simulink model "BaseEngineController_LS_112"  (Simulink 7.7)
settings: Solver=FixedStepDiscrete  StartTime=0.0  StopTime=10.0  RelTol=1e-3
PreLoadFcn:
  | try, eval([bdroot '_setup']); catch, eval('model_setup', ''); end
InitFcn:
  | try, eval([bdroot '_setup']); catch, eval('model_setup', ''); end
undefined symbols (not defined in the file): ECM, H1, H2, High, motohawk_build_version, motohawk_trunc_name, motohawk_vardec_config_group, motohawk_vardec_path, True, xD
libraries: MotoHawk_lib x1417, motohawk_control_primitives_lib x183, motohawk_engine_lib x32, simulink x21, motohawk_annotations_lib x9, AutoDoc_lib x8, simulink_extras x4, motohawk_ccp_examples_lib x1, motohawk_control_primitives_motoshare_lib x1
(part 26 of 27)

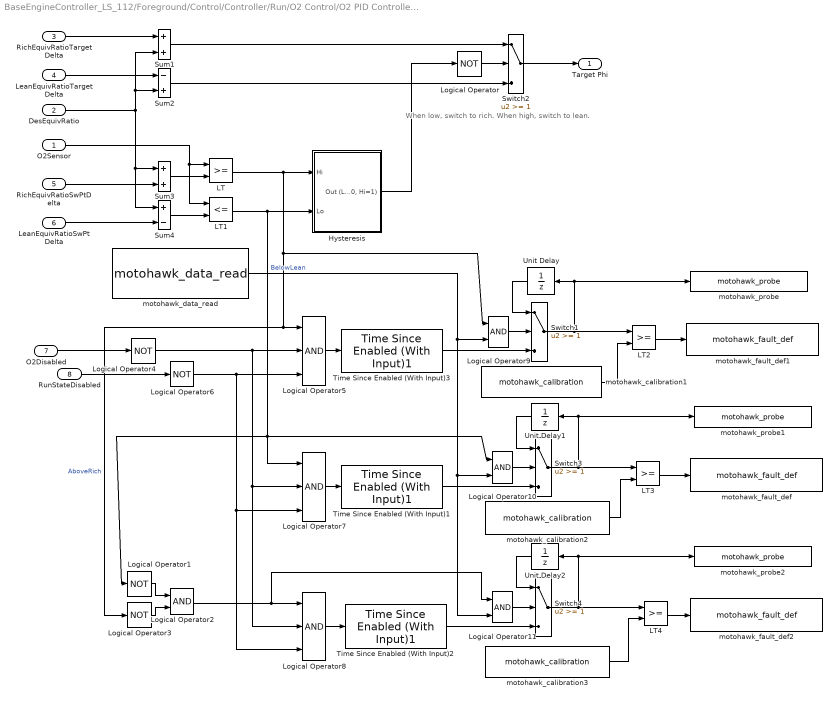
== system BaseEngineController_LS_112/Foreground/Control/Controller/Run/O2 Control/O2 PID Controller Bank A/Equivalence Ratio Perturbation ==
  note: When low, switch to rich.
      | When high, switch to lean.
  O2Sensor : Inport
  DesEquivRatio : Inport  Port=2
  RichEquivRatioTargetDelta : Inport  Port=3
  LeanEquivRatioTargetDelta : Inport  Port=4
  RichEquivRatioSwPtDelta : Inport  Port=5
  LeanEquivRatioSwPtDelta : Inport  Port=6
  O2Disabled : Inport  Port=7
  RunStateDisabled : Inport  Port=8
  Hysteresis : Subsystem
  LT{,2..4} (4 alike) : RelationalOperator  ZeroCross=off  InputSameDT=on
  LT1 : RelationalOperator  Operator=<=  ZeroCross=off  InputSameDT=on
  Logical Operator{,1,3..4,6} (5 alike) : Logic  Operator=NOT
  Logical Operator{2,9..11} (4 alike) : Logic
  Logical Operator5 : Logic  Inputs=3
  Logical Operator7 : Logic  Inputs=3
  Logical Operator8 : Logic  Inputs=3
  Sum1 : Sum  SaturateOnIntegerOverflow=on
  Sum2 : Sum  Inputs=-+  SaturateOnIntegerOverflow=on
  Sum3 : Sum  SaturateOnIntegerOverflow=on
  Sum4 : Sum  Inputs=+-  SaturateOnIntegerOverflow=on
  Switch{1..4} (4 alike) : Switch  Threshold=1  ZeroCross=off  InputSameDT=on
  Time Since Enabled (With Input)1 : motohawk_control_primitives_lib/Time Since Enabled (With Input)1  SystemSampleTime=-1  nam='O2LeanTimer_BankA'  samp_time=-1  init=0  upperlim=16000
  Time Since Enabled (With Input)2 : motohawk_control_primitives_lib/Time Since Enabled (With Input)1  SystemSampleTime=-1  nam='O2ActiveTimer_BankA'  samp_time=-1  init=0  upperlim=16000
  Time Since Enabled (With Input)3 : motohawk_control_primitives_lib/Time Since Enabled (With Input)1  SystemSampleTime=-1  nam='O2RichTimer_BankA'  samp_time=-1  init=0  upperlim=16000
  Unit Delay : UnitDelay  SampleTime=-1
  Unit Delay1 : UnitDelay  SampleTime=-1
  Unit Delay2 : UnitDelay  SampleTime=-1
  motohawk_calibration1 : MotoHawk_lib/Calibration & Probing Blocks/motohawk_calibration  nam='O2RichTimeThresh_BankA'  val=40  storage=Calibration  show_more=on  name_source=Use Parameter  data_type=Inherit from 'Default Value'  read_level=1  write_level=1  ovr_cals=on  view_as=Number  enum_struct={'Disabled', 'Enabled'}  vector_style=Wide Row  use_help_units=on  help='Time limit the O2 feedback can sit abovethe rich switch point before flagging O2FailedRich fault'  units='s'  use_header_enum=off  row_header_enum={}  col_header_enum={}  use_min_max=off  min_val=-inf  max_val=inf  use_precision=off  precision=''  gain=1  offset=0  exp=1  use_mototune_group=on  mototune_group=motohawk_vardec_path(gcb)
  motohawk_calibration2 : MotoHawk_lib/Calibration & Probing Blocks/motohawk_calibration  nam='O2LeanTimeThresh_BankA'  val=10  storage=Calibration  show_more=on  name_source=Use Parameter  data_type=Inherit from 'Default Value'  read_level=1  write_level=1  ovr_cals=on  view_as=Number  enum_struct={'Disabled', 'Enabled'}  vector_style=Wide Row  use_help_units=on  help='Time limit the O2 feedback can sit below the lean switch point before flagging O2FailedLean fault'  units='s'  use_header_enum=off  row_header_enum={}  col_header_enum={}  use_min_max=off  min_val=-inf  max_val=inf  use_precision=off  precision=''  gain=1  offset=0  exp=1  use_mototune_group=on  mototune_group=motohawk_vardec_path(gcb)
  motohawk_calibration3 : MotoHawk_lib/Calibration & Probing Blocks/motohawk_calibration  nam='O2ActiveTimeThresh_BankA'  val=40  storage=Calibration  show_more=on  name_source=Use Parameter  data_type=Inherit from 'Default Value'  read_level=1  write_level=1  ovr_cals=on  view_as=Number  enum_struct={'Disabled', 'Enabled'}  vector_style=Wide Row  use_help_units=on  help='Time limit O2 feedback can sit between rich and lean switch points before flagging O2NotActive fault'  units='s'  use_header_enum=off  row_header_enum={}  col_header_enum={}  use_min_max=off  min_val=-inf  max_val=inf  use_precision=off  precision=''  gain=1  offset=0  exp=1  use_mototune_group=on  mototune_group=motohawk_vardec_path(gcb)
  motohawk_data_read : MotoHawk_lib/Data Storage Blocks/motohawk_data_read  source=Lookup By Name  structure=Scalar  operation=Read scalar from location by index  sz_vec=4  sz_row=2  sz_col=3  typ=boolean  nam='DisableO2FaultAction'  checkNull=on  struct_inst_name='Struct1'  struct_nam='MyStruct'
  motohawk_fault_def : MotoHawk_lib/Fault Management Blocks/motohawk_fault_def  nam='O2FailedLean_BankA'  mode=Enabled  id=[]  x=25  y=50  input_suspected=on  indeterminate=off  increment_xy=on  downsample_count=1  ovr_cals=on  ovr_actions=on  show_actions=off  action1_name=''  action1_cond=(None)  action2_name=''  action2_cond=(None)  action3_name=''  action3_cond=(None)  action4_name=''  action4_cond=(None)
  motohawk_fault_def1 : MotoHawk_lib/Fault Management Blocks/motohawk_fault_def  nam='O2FailedRich_BankA'  mode=Enabled  id=[]  x=25  y=50  input_suspected=on  indeterminate=off  increment_xy=on  downsample_count=1  ovr_cals=on  ovr_actions=on  show_actions=off  action1_name=''  action1_cond=(None)  action2_name=''  action2_cond=(None)  action3_name=''  action3_cond=(None)  action4_name=''  action4_cond=(None)
  motohawk_fault_def2 : MotoHawk_lib/Fault Management Blocks/motohawk_fault_def  nam='O2NotActive_BankA'  mode=Enabled  id=[]  x=25  y=50  input_suspected=on  indeterminate=off  increment_xy=on  downsample_count=1  ovr_cals=on  ovr_actions=on  show_actions=off  action1_name=''  action1_cond=(None)  action2_name=''  action2_cond=(None)  action3_name=''  action3_cond=(None)  action4_name=''  action4_cond=(None)
  motohawk_probe : MotoHawk_lib/Calibration & Probing Blocks/motohawk_probe  nam='O2RichTime_BankA'  show_more=on  name_source=Use Parameter  read_level=1  view_as=Number  enum_struct={'Disabled', 'Enabled'}  vector_style=Wide Row  use_help_units=off  help=''  units=''  use_header_enum=off  row_header_enum={}  col_header_enum={}  use_precision=off  precision=''  gain=1  offset=0  exp=1  use_mototune_group=on  mototune_group=motohawk_vardec_path(gcb)
  motohawk_probe1 : MotoHawk_lib/Calibration & Probing Blocks/motohawk_probe  nam='O2LeanTime_BankA'  show_more=on  name_source=Use Parameter  read_level=1  view_as=Number  enum_struct={'Disabled', 'Enabled'}  vector_style=Wide Row  use_help_units=off  help=''  units=''  use_header_enum=off  row_header_enum={}  col_header_enum={}  use_precision=off  precision=''  gain=1  offset=0  exp=1  use_mototune_group=on  mototune_group=motohawk_vardec_path(gcb)
  motohawk_probe2 : MotoHawk_lib/Calibration & Probing Blocks/motohawk_probe  nam='O2NotActiveTime_BankA'  show_more=on  name_source=Use Parameter  read_level=1  view_as=Number  enum_struct={'Disabled', 'Enabled'}  vector_style=Wide Row  use_help_units=off  help=''  units=''  use_header_enum=off  row_header_enum={}  col_header_enum={}  use_precision=off  precision=''  gain=1  offset=0  exp=1  use_mototune_group=on  mototune_group=motohawk_vardec_path(gcb)
  Target Phi : Outport
  wires:
  Sum3/1 -> LT/2
  Sum4/1 -> LT1/2
  Switch2/1 -> Target Phi/1
  DesEquivRatio/1 -> Sum1/2, Sum2/2, Sum4/1, Sum3/1
  RichEquivRatioSwPtDelta/1 -> Sum3/2
  LeanEquivRatioSwPtDelta/1 -> Sum4/2
  Sum2/1 -> Switch2/3
  Sum1/1 -> Switch2/1
  LeanEquivRatioTargetDelta/1 -> Sum2/1
  RichEquivRatioTargetDelta/1 -> Sum1/1
  LT/1 -> Hysteresis/1(Hi), Logical Operator5/1, Logical Operator3/1, Logical Operator9/1  "AboveRich"
  LT1/1 -> Hysteresis/2(Lo), Logical Operator1/1, Logical Operator7/1, Logical Operator10/1  "BelowLean"
  Hysteresis/1("Out (Lo=0, Hi=1)") -> Logical Operator/1
  O2Sensor/1 -> LT1/1, LT/1
  Logical Operator/1 -> Switch2/2
  motohawk_calibration1/1 -> LT2/2
  LT2/1 -> motohawk_fault_def1/1
  LT3/1 -> motohawk_fault_def/1
  motohawk_calibration2/1 -> LT3/2
  LT4/1 -> motohawk_fault_def2/1
  motohawk_calibration3/1 -> LT4/2
  Logical Operator1/1 -> Logical Operator2/1
  Logical Operator3/1 -> Logical Operator2/2
  Logical Operator4/1 -> Logical Operator5/2, Logical Operator7/2, Logical Operator8/2
  O2Disabled/1 -> Logical Operator4/1
  RunStateDisabled/1 -> Logical Operator6/1
  Logical Operator6/1 -> Logical Operator5/3, Logical Operator7/3, Logical Operator8/3
  Logical Operator2/1 -> Logical Operator8/1, Logical Operator11/1
  Logical Operator5/1 -> Time Since Enabled (With Input)3/1
  Logical Operator7/1 -> Time Since Enabled (With Input)1/1
  Logical Operator8/1 -> Time Since Enabled (With Input)2/1
  Unit Delay/1 -> Switch1/1
  Time Since Enabled (With Input)3/1 -> Switch1/3
  Switch1/1 -> LT2/1, Unit Delay/1, motohawk_probe/1
  Logical Operator9/1 -> Switch1/2
  motohawk_data_read/1 -> Logical Operator9/2, Logical Operator10/2, Logical Operator11/2
  Unit Delay1/1 -> Switch3/1
  Switch3/1 -> LT3/1, Unit Delay1/1, motohawk_probe1/1
  Logical Operator10/1 -> Switch3/2
  Time Since Enabled (With Input)1/1 -> Switch3/3
  Unit Delay2/1 -> Switch4/1
  Switch4/1 -> LT4/1, Unit Delay2/1, motohawk_probe2/1
  Logical Operator11/1 -> Switch4/2
  Time Since Enabled (With Input)2/1 -> Switch4/3

== system BaseEngineController_LS_112/Foreground/Control/Controller/Run/O2 Control/O2 PID Controller Bank B/Closed-Loop O2 PID Controller ==
  O2Sensor : Inport
  TargetEquivRatio : Inport  Port=2
  ErrorGain : Inport  Port=3
  PGain : Inport  Port=4
  IGain : Inport  Port=5
  DGain : Inport  Port=6
  ITermUpperLimit : Inport  Port=7
  ITermLowerLimit : Inport  Port=8
  OutUpperLimit : Inport  Port=9
  OutLowerLimit : Inport  Port=10
  Reset : Inport  Port=11
  Constant : Constant  Value=0  OutDataTypeStr=Inherit: Inherit via back propagation
  Convert to Fuel Multiplier : Constant  OutDataTypeStr=Inherit: Inherit via back propagation
  Saturation : motohawk_control_primitives_lib/Saturation  SystemSampleTime=-1
  Sum : Sum  Inputs=++|  SaturateOnIntegerOverflow=on  InputSameDT=on
  Universal PID : motohawk_control_primitives_lib/Universal PID  Description=|  SystemSampleTime=-1  samp_time=.005
      | /* Name: ErrorGain Unit:mult ClassID:VAR StorageID:FLASH Access:RW4+RW3+NA2+NA1 TypeID:UINT4                   
      |    Gain:0.000000001 Min:0.000000000 Max:4.000000000 Format:10.9 UpdateID:REMOTE Help:"This gain is applied to "
      |    "the error term before it is used to calculate the P, I and D terms." VardecSig:6C */                       
      |                                                                                                                
      | /* Name: ITermLowerLim Unit:0 ClassID:VAR StorageID:FLASH Access:RW4+RW3+NA2+NA1 TypeID:SINT2 Gain:0.1         
      |    Min:-3276.8 Max:3276.7 Format:5.1 UpdateID:REMOTE Help:"Lower limit on the I-term value." VardecSig:6C */   
      |                                                                                                                
      | /* Name: ITermUpperLim ClassID:VAR StorageID:FLASH Access:RW4+RW3+NA2+NA1 TypeID:SINT2 Gain:0.1 Min:-3276.8    
      |    Max:3276.7 Format:5.1 UpdateID:REMOTE Help:"Upper limit on I-term value." VardecSig:6C */                   
      |                                                                                                                
      | /* Name: PIDOutLowerLim ClassID:VAR StorageID:FLASH Access:RW4+RW3+NA2+NA1 TypeID:SINT2 Gain:0.1               
      |    Min:-3276.8 Max:3276.7 Format:5.1 UpdateID:REMOTE Help:"Lower limit on PID output." VardecSig:6C */         
      |                                                                                                                
      | /* Name: PIDOutUpperLim ClassID:VAR StorageID:FLASH Access:RW4+RW3+NA2+NA1 TypeID:SINT2 Gain:0.1               
      |    Min:-3276.8 Max:3276.7 Format:3.1 UpdateID:REMOTE Help:"Upper limit on PID output." VardecSig:6C */
  motohawk_probe : MotoHawk_lib/Calibration & Probing Blocks/motohawk_probe  nam='LiquidO2Control_PTerm_BankB'  show_more=on  name_source=Use Parameter  read_level=1  view_as=Number  enum_struct={'Disabled', 'Enabled'}  vector_style=Wide Row  use_help_units=on  help='Closed-loop O2 control P-Term'  units='mult'  use_header_enum=off  row_header_enum={}  col_header_enum={}  use_precision=off  precision=''  gain=1  offset=0  exp=1  use_mototune_group=on  mototune_group=motohawk_vardec_path(gcb)
  motohawk_probe1 : MotoHawk_lib/Calibration & Probing Blocks/motohawk_probe  nam='LiquidO2Control_ITerm_BankB'  show_more=on  name_source=Use Parameter  read_level=1  view_as=Number  enum_struct={'Disabled', 'Enabled'}  vector_style=Wide Row  use_help_units=on  help='Closed-loop O2 control I-Term'  units='mult'  use_header_enum=off  row_header_enum={}  col_header_enum={}  use_precision=off  precision=''  gain=1  offset=0  exp=1  use_mototune_group=on  mototune_group=motohawk_vardec_path(gcb)
  motohawk_probe2 : MotoHawk_lib/Calibration & Probing Blocks/motohawk_probe  nam='LiquidO2Control_DTerm_BankB'  show_more=on  name_source=Use Parameter  read_level=1  view_as=Number  enum_struct={'Disabled', 'Enabled'}  vector_style=Wide Row  use_help_units=on  help='Closed-loop O2 control D-Term, for bank'  units='mult'  use_header_enum=off  row_header_enum={}  col_header_enum={}  use_precision=off  precision=''  gain=1  offset=0  exp=1  use_mototune_group=on  mototune_group=motohawk_vardec_path(gcb)
  motohawk_probe3 : MotoHawk_lib/Calibration & Probing Blocks/motohawk_probe  nam='LiquidO2Control_ErrorTerm_BankB'  show_more=on  name_source=Use Parameter  read_level=1  view_as=Number  enum_struct={'Disabled', 'Enabled'}  vector_style=Wide Row  use_help_units=on  help='Closed-loop O2 control error-term, for bank'  units='mult'  use_header_enum=off  row_header_enum={}  col_header_enum={}  use_precision=off  precision=''  gain=1  offset=0  exp=1  use_mototune_group=on  mototune_group=motohawk_vardec_path(gcb)
  Multiplier : Outport
  ITerm : Outport  Port=2
  wires:
  Reset/1 -> Universal PID/10
  Universal PID/3 -> motohawk_probe/1
  Universal PID/4 -> motohawk_probe1/1, ITerm/1
  Constant/1 -> Universal PID/7
  Universal PID/5 -> motohawk_probe2/1
  Saturation/1 -> Multiplier/1
  O2Sensor/1 -> Universal PID/1
  TargetEquivRatio/1 -> Universal PID/2
  ErrorGain/1 -> Universal PID/3
  PGain/1 -> Universal PID/4
  IGain/1 -> Universal PID/5
  DGain/1 -> Universal PID/6
  OutUpperLimit/1 -> Saturation/3
  Convert to Fuel Multiplier/1 -> Sum/1
  Universal PID/1 -> Sum/2
  Sum/1 -> Saturation/1
  ITermUpperLimit/1 -> Universal PID/9
  ITermLowerLimit/1 -> Universal PID/8
  OutLowerLimit/1 -> Saturation/2
  Universal PID/2 -> motohawk_probe3/1

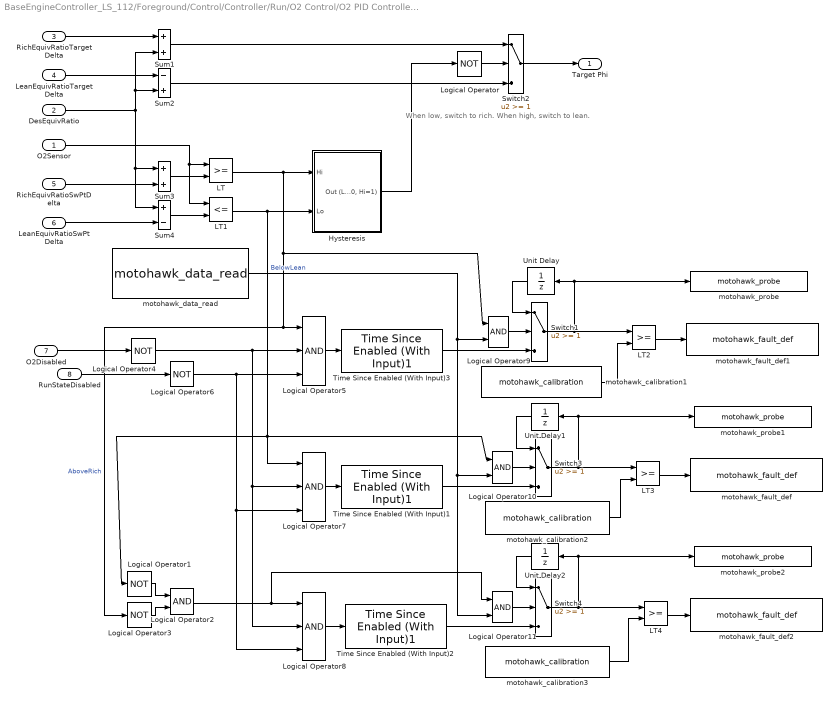
== system BaseEngineController_LS_112/Foreground/Control/Controller/Run/O2 Control/O2 PID Controller Bank B/Equivalence Ratio Perturbation ==
  note: When low, switch to rich.
      | When high, switch to lean.
  O2Sensor : Inport
  DesEquivRatio : Inport  Port=2
  RichEquivRatioTargetDelta : Inport  Port=3
  LeanEquivRatioTargetDelta : Inport  Port=4
  RichEquivRatioSwPtDelta : Inport  Port=5
  LeanEquivRatioSwPtDelta : Inport  Port=6
  O2Disabled : Inport  Port=7
  RunStateDisabled : Inport  Port=8
  Hysteresis : Subsystem
  LT{,2..4} (4 alike) : RelationalOperator  ZeroCross=off  InputSameDT=on
  LT1 : RelationalOperator  Operator=<=  ZeroCross=off  InputSameDT=on
  Logical Operator{,1,3..4,6} (5 alike) : Logic  Operator=NOT
  Logical Operator{2,9..11} (4 alike) : Logic
  Logical Operator5 : Logic  Inputs=3
  Logical Operator7 : Logic  Inputs=3
  Logical Operator8 : Logic  Inputs=3
  Sum1 : Sum  SaturateOnIntegerOverflow=on
  Sum2 : Sum  Inputs=-+  SaturateOnIntegerOverflow=on
  Sum3 : Sum  SaturateOnIntegerOverflow=on
  Sum4 : Sum  Inputs=+-  SaturateOnIntegerOverflow=on
  Switch{1..4} (4 alike) : Switch  Threshold=1  ZeroCross=off  InputSameDT=on
  Time Since Enabled (With Input)1 : motohawk_control_primitives_lib/Time Since Enabled (With Input)1  SystemSampleTime=-1  nam='O2LeanTimer_BankB'  samp_time=-1  init=0  upperlim=16000
  Time Since Enabled (With Input)2 : motohawk_control_primitives_lib/Time Since Enabled (With Input)1  SystemSampleTime=-1  nam='O2ActiveTimer_BankB'  samp_time=-1  init=0  upperlim=16000
  Time Since Enabled (With Input)3 : motohawk_control_primitives_lib/Time Since Enabled (With Input)1  SystemSampleTime=-1  nam='O2RichTimer_BankB'  samp_time=-1  init=0  upperlim=16000
  Unit Delay : UnitDelay  SampleTime=-1
  Unit Delay1 : UnitDelay  SampleTime=-1
  Unit Delay2 : UnitDelay  SampleTime=-1
  motohawk_calibration1 : MotoHawk_lib/Calibration & Probing Blocks/motohawk_calibration  nam='O2RichTimeThresh_BankB'  val=40  storage=Calibration  show_more=on  name_source=Use Parameter  data_type=Inherit from 'Default Value'  read_level=1  write_level=1  ovr_cals=on  view_as=Number  enum_struct={'Disabled', 'Enabled'}  vector_style=Wide Row  use_help_units=on  help='Time limit the O2 feedback can sit abovethe rich switch point before flagging O2FailedRich fault'  units='s'  use_header_enum=off  row_header_enum={}  col_header_enum={}  use_min_max=off  min_val=-inf  max_val=inf  use_precision=off  precision=''  gain=1  offset=0  exp=1  use_mototune_group=on  mototune_group=motohawk_vardec_path(gcb)
  motohawk_calibration2 : MotoHawk_lib/Calibration & Probing Blocks/motohawk_calibration  nam='O2LeanTimeThresh_BankB'  val=10  storage=Calibration  show_more=on  name_source=Use Parameter  data_type=Inherit from 'Default Value'  read_level=1  write_level=1  ovr_cals=on  view_as=Number  enum_struct={'Disabled', 'Enabled'}  vector_style=Wide Row  use_help_units=on  help='Time limit the O2 feedback can sit below the lean switch point before flagging O2FailedLean fault'  units='s'  use_header_enum=off  row_header_enum={}  col_header_enum={}  use_min_max=off  min_val=-inf  max_val=inf  use_precision=off  precision=''  gain=1  offset=0  exp=1  use_mototune_group=on  mototune_group=motohawk_vardec_path(gcb)
  motohawk_calibration3 : MotoHawk_lib/Calibration & Probing Blocks/motohawk_calibration  nam='O2ActiveTimeThresh_BankB'  val=40  storage=Calibration  show_more=on  name_source=Use Parameter  data_type=Inherit from 'Default Value'  read_level=1  write_level=1  ovr_cals=on  view_as=Number  enum_struct={'Disabled', 'Enabled'}  vector_style=Wide Row  use_help_units=on  help='Time limit O2 feedback can sit between rich and lean switch points before flagging O2NotActive fault'  units='s'  use_header_enum=off  row_header_enum={}  col_header_enum={}  use_min_max=off  min_val=-inf  max_val=inf  use_precision=off  precision=''  gain=1  offset=0  exp=1  use_mototune_group=on  mototune_group=motohawk_vardec_path(gcb)
  motohawk_data_read : MotoHawk_lib/Data Storage Blocks/motohawk_data_read  source=Lookup By Name  structure=Scalar  operation=Read scalar from location by index  sz_vec=4  sz_row=2  sz_col=3  typ=boolean  nam='DisableO2FaultAction'  checkNull=on  struct_inst_name='Struct1'  struct_nam='MyStruct'
  motohawk_fault_def : MotoHawk_lib/Fault Management Blocks/motohawk_fault_def  nam='O2FailedLean_BankB'  mode=Enabled  id=[]  x=25  y=50  input_suspected=on  indeterminate=off  increment_xy=on  downsample_count=1  ovr_cals=on  ovr_actions=on  show_actions=off  action1_name=''  action1_cond=(None)  action2_name=''  action2_cond=(None)  action3_name=''  action3_cond=(None)  action4_name=''  action4_cond=(None)
  motohawk_fault_def1 : MotoHawk_lib/Fault Management Blocks/motohawk_fault_def  nam='O2FailedRich_BankB'  mode=Enabled  id=[]  x=25  y=50  input_suspected=on  indeterminate=off  increment_xy=on  downsample_count=1  ovr_cals=on  ovr_actions=on  show_actions=off  action1_name=''  action1_cond=(None)  action2_name=''  action2_cond=(None)  action3_name=''  action3_cond=(None)  action4_name=''  action4_cond=(None)
  motohawk_fault_def2 : MotoHawk_lib/Fault Management Blocks/motohawk_fault_def  nam='O2NotActive_BankB'  mode=Enabled  id=[]  x=25  y=50  input_suspected=on  indeterminate=off  increment_xy=on  downsample_count=1  ovr_cals=on  ovr_actions=on  show_actions=off  action1_name=''  action1_cond=(None)  action2_name=''  action2_cond=(None)  action3_name=''  action3_cond=(None)  action4_name=''  action4_cond=(None)
  motohawk_probe : MotoHawk_lib/Calibration & Probing Blocks/motohawk_probe  nam='O2RichTime_BankB'  show_more=on  name_source=Use Parameter  read_level=1  view_as=Number  enum_struct={'Disabled', 'Enabled'}  vector_style=Wide Row  use_help_units=off  help=''  units=''  use_header_enum=off  row_header_enum={}  col_header_enum={}  use_precision=off  precision=''  gain=1  offset=0  exp=1  use_mototune_group=on  mototune_group=motohawk_vardec_path(gcb)
  motohawk_probe1 : MotoHawk_lib/Calibration & Probing Blocks/motohawk_probe  nam='O2LeanTime_BankB'  show_more=on  name_source=Use Parameter  read_level=1  view_as=Number  enum_struct={'Disabled', 'Enabled'}  vector_style=Wide Row  use_help_units=off  help=''  units=''  use_header_enum=off  row_header_enum={}  col_header_enum={}  use_precision=off  precision=''  gain=1  offset=0  exp=1  use_mototune_group=on  mototune_group=motohawk_vardec_path(gcb)
  motohawk_probe2 : MotoHawk_lib/Calibration & Probing Blocks/motohawk_probe  nam='O2NotActiveTime_BankB'  show_more=on  name_source=Use Parameter  read_level=1  view_as=Number  enum_struct={'Disabled', 'Enabled'}  vector_style=Wide Row  use_help_units=off  help=''  units=''  use_header_enum=off  row_header_enum={}  col_header_enum={}  use_precision=off  precision=''  gain=1  offset=0  exp=1  use_mototune_group=on  mototune_group=motohawk_vardec_path(gcb)
  Target Phi : Outport
  wires:
  Sum3/1 -> LT/2
  Sum4/1 -> LT1/2
  Switch2/1 -> Target Phi/1
  DesEquivRatio/1 -> Sum1/2, Sum2/2, Sum4/1, Sum3/1
  RichEquivRatioSwPtDelta/1 -> Sum3/2
  LeanEquivRatioSwPtDelta/1 -> Sum4/2
  Sum2/1 -> Switch2/3
  Sum1/1 -> Switch2/1
  LeanEquivRatioTargetDelta/1 -> Sum2/1
  RichEquivRatioTargetDelta/1 -> Sum1/1
  LT/1 -> Hysteresis/1(Hi), Logical Operator5/1, Logical Operator3/1, Logical Operator9/1  "AboveRich"
  LT1/1 -> Hysteresis/2(Lo), Logical Operator1/1, Logical Operator7/1, Logical Operator10/1  "BelowLean"
  Hysteresis/1("Out (Lo=0, Hi=1)") -> Logical Operator/1
  O2Sensor/1 -> LT1/1, LT/1
  Logical Operator/1 -> Switch2/2
  motohawk_calibration1/1 -> LT2/2
  LT2/1 -> motohawk_fault_def1/1
  LT3/1 -> motohawk_fault_def/1
  motohawk_calibration2/1 -> LT3/2
  LT4/1 -> motohawk_fault_def2/1
  motohawk_calibration3/1 -> LT4/2
  Logical Operator1/1 -> Logical Operator2/1
  Logical Operator3/1 -> Logical Operator2/2
  Logical Operator4/1 -> Logical Operator5/2, Logical Operator7/2, Logical Operator8/2
  O2Disabled/1 -> Logical Operator4/1
  RunStateDisabled/1 -> Logical Operator6/1
  Logical Operator6/1 -> Logical Operator5/3, Logical Operator7/3, Logical Operator8/3
  Logical Operator2/1 -> Logical Operator8/1, Logical Operator11/1
  Logical Operator5/1 -> Time Since Enabled (With Input)3/1
  Logical Operator7/1 -> Time Since Enabled (With Input)1/1
  Logical Operator8/1 -> Time Since Enabled (With Input)2/1
  Unit Delay/1 -> Switch1/1
  Time Since Enabled (With Input)3/1 -> Switch1/3
  Switch1/1 -> LT2/1, Unit Delay/1, motohawk_probe/1
  Logical Operator9/1 -> Switch1/2
  motohawk_data_read/1 -> Logical Operator9/2, Logical Operator10/2, Logical Operator11/2
  Unit Delay1/1 -> Switch3/1
  Switch3/1 -> LT3/1, Unit Delay1/1, motohawk_probe1/1
  Logical Operator10/1 -> Switch3/2
  Time Since Enabled (With Input)1/1 -> Switch3/3
  Unit Delay2/1 -> Switch4/1
  Switch4/1 -> LT4/1, Unit Delay2/1, motohawk_probe2/1
  Logical Operator11/1 -> Switch4/2
  Time Since Enabled (With Input)2/1 -> Switch4/3

== system BaseEngineController_LS_112/Foreground/Control/Controller/Stall/FAN Control/Hysterisis/Hysteresis ==
  note: Hi & !Lo => Hi
      | Lo & !Hi => Lo
      | Otherwise, Hold
  Hi : Inport
  Lo : Inport  Port=2
  Combinatorial  Logic : CombinatorialLogic  TruthTable=[0 0;0 1;1 1;0 0]
  Demux : Demux  Outputs=2
  Mux : Mux  Inputs=2
  Switch1 : Switch  Threshold=0.5  SaturateOnIntegerOverflow=on  InputSameDT=on
  Unit Delay : UnitDelay  SampleTime=-1
  "Out (Lo=0, Hi=1)" : Outport
  wires:
  Mux/1 -> Combinatorial  Logic/1
  Combinatorial  Logic/1 -> Demux/1
  Demux/1 -> Switch1/1
  Demux/2 -> Switch1/2
  Unit Delay/1 -> Switch1/3
  Switch1/1 -> Unit Delay/1, "Out (Lo=0, Hi=1)"/1
  Hi/1 -> Mux/1
  Lo/1 -> Mux/2

== system BaseEngineController_LS_112/Foreground/Control/Controller/Stall/FAN Control/Hysterisis1/Hysteresis ==
  note: Hi & !Lo => Hi
      | Lo & !Hi => Lo
      | Otherwise, Hold
  Hi : Inport
  Lo : Inport  Port=2
  Combinatorial  Logic : CombinatorialLogic  TruthTable=[0 0;0 1;1 1;0 0]
  Demux : Demux  Outputs=2
  Mux : Mux  Inputs=2
  Switch1 : Switch  Threshold=0.5  SaturateOnIntegerOverflow=on  InputSameDT=on
  Unit Delay : UnitDelay  SampleTime=-1
  "Out (Lo=0, Hi=1)" : Outport
  wires:
  Mux/1 -> Combinatorial  Logic/1
  Combinatorial  Logic/1 -> Demux/1
  Demux/1 -> Switch1/1
  Demux/2 -> Switch1/2
  Unit Delay/1 -> Switch1/3
  Switch1/1 -> Unit Delay/1, "Out (Lo=0, Hi=1)"/1
  Hi/1 -> Mux/1
  Lo/1 -> Mux/2

== system BaseEngineController_LS_112/Foreground/Control/Controller/Stall/FAN Control/Hysterisis2/Hysteresis ==
  note: Hi & !Lo => Hi
      | Lo & !Hi => Lo
      | Otherwise, Hold
  Hi : Inport
  Lo : Inport  Port=2
  Combinatorial  Logic : CombinatorialLogic  TruthTable=[0 0;0 1;1 1;0 0]
  Demux : Demux  Outputs=2
  Mux : Mux  Inputs=2
  Switch1 : Switch  Threshold=0.5  SaturateOnIntegerOverflow=on  InputSameDT=on
  Unit Delay : UnitDelay  SampleTime=-1
  "Out (Lo=0, Hi=1)" : Outport
  wires:
  Mux/1 -> Combinatorial  Logic/1
  Combinatorial  Logic/1 -> Demux/1
  Demux/1 -> Switch1/1
  Demux/2 -> Switch1/2
  Unit Delay/1 -> Switch1/3
  Switch1/1 -> Unit Delay/1, "Out (Lo=0, Hi=1)"/1
  Hi/1 -> Mux/1
  Lo/1 -> Mux/2

== system BaseEngineController_LS_112/Foreground/Control/Diagnostics/MISFIRE/MisfireDiagSub/MisfireDiagFunc/DetermineMisfire ==
  Compare To Constant : simulink/Logic and Bit Operations/Compare To Constant  SystemSampleTime=-1  relop=>  const=0  LogicOutDataTypeMode=uint8
  DetermineCylinder : Subsystem
  Logical Operator1 : Logic  AllPortsSameDT=off  OutDataTypeStr=boolean
  Product : Product  RndMeth=Zero
  Relational Operator1 : RelationalOperator  Operator=<=  OutDataTypeStr=boolean
  Rising Edge : motohawk_control_primitives_lib/Rising Edge  SystemSampleTime=-1
  SetHardFault : Subsystem
  Sum : Sum  Inputs=|+-
  motohawk_calibration1 : MotoHawk_lib/Calibration & Probing Blocks/motohawk_calibration  nam='MisfireDiag_HardMisfireThreshold'  val=50  storage=Calibration  show_more=off  name_source=Use Parameter  data_type=Inherit from 'Default Value'  read_level=1  write_level=1  ovr_cals=on  view_as=Number  enum_struct={'Disabled', 'Enabled'}  vector_style=Wide Row  use_help_units=off  help=''  units=''  use_header_enum=off  row_header_enum={}  col_header_enum={}  use_min_max=off  min_val=-inf  max_val=inf  use_precision=off  precision=''  gain=1  offset=0  exp=1  use_mototune_group=off  mototune_group=motohawk_vardec_path(gcb)
  motohawk_data_read : MotoHawk_lib/Data Storage Blocks/motohawk_data_read  source=Lookup By Name  structure=Vector  operation=Read scalar from location by index  sz_vec=8  sz_row=2  sz_col=3  typ=uint16  nam='MisfireDiag_StartRPM'  checkNull=on  struct_inst_name='MyData'  struct_nam='MyStruct'
  motohawk_data_read1 : MotoHawk_lib/Data Storage Blocks/motohawk_data_read  source=Lookup By Name  structure=Vector  operation=Read scalar from location by index  sz_vec=8  sz_row=2  sz_col=3  typ=uint16  nam='MisfireDiag_StopRPM'  checkNull=on  struct_inst_name='MyData'  struct_nam='MyStruct'
  motohawk_data_read2 : MotoHawk_lib/Data Storage Blocks/motohawk_data_read  source=Lookup By Name  structure=Vector  operation=Read entire data structure at once  sz_vec=8  sz_row=2  sz_col=3  typ=boolean  nam='MisfireDiag_RPMDR'  checkNull=on  struct_inst_name='MyData'  struct_nam='MyStruct'
  wires:
  motohawk_data_read2/1 -> Rising Edge/1
  Sum/1 -> [RPMDelta]
  motohawk_data_read1/1 -> Sum/1
  motohawk_data_read/1 -> Sum/2
  [RPMDelta] -> Relational Operator1/1
  motohawk_calibration1/1 -> Relational Operator1/2
  Rising Edge/1 -> [RPMDR_Rising]
  Logical Operator1/1 -> Product/2
  [RPMDR_Rising] -> DetermineCylinder/1(ArrayIn)
  DetermineCylinder/1(CylinderNum) -> motohawk_data_read1/1, motohawk_data_read/1, Compare To Constant/1, Product/1
  Relational Operator1/1 -> Logical Operator1/1
  Compare To Constant/1 -> Logical Operator1/2
  Product/1 -> SetHardFault/1(CylNum)

== system BaseEngineController_LS_112/Foreground/Control/Diagnostics/MISFIRE/MisfireDiagSub/MisfireDiagFunc/StoreRPMData ==
  DetermineCylinder : Subsystem
  DetermineCylinder1 : Subsystem
  EncoderAngleArb : Subsystem
  Gain : Gain  Gain=16
  Gain1 : Gain  Gain=16
  LatchForAverage : Subsystem
  LatchForAverage1 : Subsystem
  Logical Operator : Logic  AllPortsSameDT=off  OutDataTypeStr=boolean
  Logical Operator1 : Logic  AllPortsSameDT=off  OutDataTypeStr=boolean
  Logical Operator2 : Logic  Operator=OR  Inputs=1  AllPortsSameDT=off  OutDataTypeStr=boolean
  Logical Operator3 : Logic  Operator=OR  Inputs=1  AllPortsSameDT=off  OutDataTypeStr=boolean
  Relational Operator : RelationalOperator  Operator=<=  OutDataTypeStr=boolean
  Relational Operator1 : RelationalOperator  OutDataTypeStr=boolean
  Relational Operator2 : RelationalOperator  Operator=<=  OutDataTypeStr=boolean
  Relational Operator3 : RelationalOperator  OutDataTypeStr=boolean
  StoreRPMStart : Subsystem  TreatAsAtomicUnit=on
  StoreRPMStart1 : Subsystem  TreatAsAtomicUnit=on
  Sum : Sum  Inputs=|++
  Sum1 : Sum  Inputs=+-|
  Sum2 : Sum  Inputs=|++
  Sum3 : Sum  Inputs=+-|
  motohawk_calibration : MotoHawk_lib/Calibration & Probing Blocks/motohawk_calibration  nam='MisfireDiag_StartAngles'  val=[0,0,0,0,0,0,0,0]  storage=Calibration  show_more=on  name_source=Use Parameter  data_type=uint16  read_level=1  write_level=1  ovr_cals=on  view_as=Number  enum_struct={'Disabled', 'Enabled'}  vector_style=Wide Row  use_help_units=off  help=''  units=''  use_header_enum=off  row_header_enum={}  col_header_enum={}  use_min_max=off  min_val=-inf  max_val=inf  use_precision=off  precision=''  gain=1  offset=0  exp=1  use_mototune_group=off  mototune_group=motohawk_vardec_path(gcb)
  motohawk_calibration1 : MotoHawk_lib/Calibration & Probing Blocks/motohawk_calibration  nam='MisfireDiag_StopAngles'  val=[0,0,0,0,0,0,0,0]  storage=Calibration  show_more=on  name_source=Use Parameter  data_type=uint16  read_level=1  write_level=1  ovr_cals=on  view_as=Number  enum_struct={'Disabled', 'Enabled'}  vector_style=Wide Row  use_help_units=off  help=''  units=''  use_header_enum=off  row_header_enum={}  col_header_enum={}  use_min_max=off  min_val=-inf  max_val=inf  use_precision=off  precision=''  gain=1  offset=0  exp=1  use_mototune_group=off  mototune_group=motohawk_vardec_path(gcb)
  motohawk_calibration2 : MotoHawk_lib/Calibration & Probing Blocks/motohawk_calibration  nam='MisfireDiag_AngleHyst'  val=4  storage=Calibration  show_more=on  name_source=Use Parameter  data_type=uint16  read_level=1  write_level=1  ovr_cals=on  view_as=Number  enum_struct={'Disabled', 'Enabled'}  vector_style=Wide Row  use_help_units=off  help=''  units=''  use_header_enum=off  row_header_enum={}  col_header_enum={}  use_min_max=off  min_val=-inf  max_val=inf  use_precision=off  precision=''  gain=1  offset=0  exp=1  use_mototune_group=off  mototune_group=motohawk_vardec_path(gcb)
  motohawk_probe : MotoHawk_lib/Calibration & Probing Blocks/motohawk_probe  nam='MisfireDiag_EncoderAngle'  show_more=off  name_source=Use Parameter  read_level=1  view_as=Number  enum_struct={'Disabled', 'Enabled'}  vector_style=Wide Row  use_help_units=off  help=''  units=''  use_header_enum=off  row_header_enum={}  col_header_enum={}  use_precision=off  precision=''  gain=1  offset=0  exp=1  use_mototune_group=off  mototune_group=motohawk_vardec_path(gcb)
  motohawk_probe3 : MotoHawk_lib/Calibration & Probing Blocks/motohawk_probe  nam='MisfireDiag_AverageStartRPMDR'  show_more=off  name_source=Use Parameter  read_level=1  view_as=Number  enum_struct={'Disabled', 'Enabled'}  vector_style=Wide Row  use_help_units=off  help=''  units=''  use_header_enum=off  row_header_enum={}  col_header_enum={}  use_precision=off  precision=''  gain=1  offset=0  exp=1  use_mototune_group=off  mototune_group=motohawk_vardec_path(gcb)
  motohawk_probe4 : MotoHawk_lib/Calibration & Probing Blocks/motohawk_probe  nam='MisfireDiag_AverageStartRPM'  show_more=off  name_source=Use Parameter  read_level=1  view_as=Number  enum_struct={'Disabled', 'Enabled'}  vector_style=Wide Row  use_help_units=off  help=''  units=''  use_header_enum=off  row_header_enum={}  col_header_enum={}  use_precision=off  precision=''  gain=1  offset=0  exp=1  use_mototune_group=off  mototune_group=motohawk_vardec_path(gcb)
  motohawk_probe5 : MotoHawk_lib/Calibration & Probing Blocks/motohawk_probe  nam='MisfireDiag_AverageStopRPMDR'  show_more=off  name_source=Use Parameter  read_level=1  view_as=Number  enum_struct={'Disabled', 'Enabled'}  vector_style=Wide Row  use_help_units=off  help=''  units=''  use_header_enum=off  row_header_enum={}  col_header_enum={}  use_precision=off  precision=''  gain=1  offset=0  exp=1  use_mototune_group=off  mototune_group=motohawk_vardec_path(gcb)
  motohawk_probe6 : MotoHawk_lib/Calibration & Probing Blocks/motohawk_probe  nam='MisfireDiag_AverageStopRPM'  show_more=off  name_source=Use Parameter  read_level=1  view_as=Number  enum_struct={'Disabled', 'Enabled'}  vector_style=Wide Row  use_help_units=off  help=''  units=''  use_header_enum=off  row_header_enum={}  col_header_enum={}  use_precision=off  precision=''  gain=1  offset=0  exp=1  use_mototune_group=off  mototune_group=motohawk_vardec_path(gcb)
  wires:
  motohawk_calibration/1 -> Gain/1
  EncoderAngleArb/1(EncoderAngle_116) -> [EncoderAngle], motohawk_probe/1
  motohawk_calibration2/1 -> [EncoderAngleHyst]
  Gain/1 -> Sum1/1, Sum/2
  [EncoderAngleHyst] -> Sum/1
  [EncoderAngleHyst] -> Sum1/2
  Sum/1 -> Relational Operator/1
  Sum1/1 -> Relational Operator1/1
  [EncoderAngle] -> Relational Operator/2
  [EncoderAngle] -> Relational Operator1/2
  Relational Operator1/1 -> Logical Operator/2
  Relational Operator/1 -> Logical Operator/1
  Gain1/1 -> Sum3/1, Sum2/2
  [EncoderAngleHyst] -> Sum2/1
  [EncoderAngleHyst] -> Sum3/2
  Sum2/1 -> Relational Operator2/1
  Sum3/1 -> Relational Operator3/1
  [EncoderAngle] -> Relational Operator2/2
  [EncoderAngle] -> Relational Operator3/2
  Relational Operator3/1 -> Logical Operator1/2
  Relational Operator2/1 -> Logical Operator1/1
  motohawk_calibration1/1 -> Gain1/1
  Logical Operator/1 -> Logical Operator2/1, DetermineCylinder/1(ArrayIn)
  Logical Operator1/1 -> Logical Operator3/1, DetermineCylinder1/1(ArrayIn)
  Logical Operator2/1 -> LatchForAverage/1(Enbl)
  DetermineCylinder/1(CylinderNum) -> StoreRPMStart/2(CylinderNum)
  LatchForAverage/1(AverageRPMDR) -> StoreRPMStart/Enable, motohawk_probe3/1
  LatchForAverage/2(AverageRPM) -> StoreRPMStart/1(AverageRPM), motohawk_probe4/1
  DetermineCylinder1/1(CylinderNum) -> StoreRPMStart1/2(CylinderNum)
  LatchForAverage1/1(AverageRPMDR) -> StoreRPMStart1/Enable, motohawk_probe5/1
  LatchForAverage1/2(AverageRPM) -> StoreRPMStart1/1(AverageRPM), motohawk_probe6/1
  Logical Operator3/1 -> LatchForAverage1/1(Enbl)

== system BaseEngineController_LS_112/Foreground/Control/VirtualSensors/LoadBasedCalcs/Engine Steady-State Flag/Inc_DecFilterSelect1/DecreasingFilter ==
  Enable : EnablePort
  motohawk_calibration2 : MotoHawk_lib/Calibration & Probing Blocks/motohawk_calibration  nam=[nam 'DecFiltC']  val=1.25  storage=Calibration  show_more=on  name_source=Use Parameter  data_type=Inherit from 'Default Value'  read_level=1  write_level=1  ovr_cals=on  view_as=Number  enum_struct={'Disabled', 'Enabled'}  vector_style=Wide Row  use_help_units=on  help='Filter time constant for a decreasing signal.'  units='sec'  use_header_enum=off  row_header_enum={}  col_header_enum={}  use_min_max=off  min_val=-inf  max_val=inf  use_precision=off  precision=''  gain=1  offset=0  exp=1  use_mototune_group=on  mototune_group=grp_cal
  Out1 : Outport  InitialOutput=.005
  wires:
  motohawk_calibration2/1 -> Out1/1

== system BaseEngineController_LS_112/Foreground/Control/VirtualSensors/LoadBasedCalcs/Engine Steady-State Flag/Inc_DecFilterSelect1/IncreasingFilter ==
  Enable : EnablePort
  motohawk_calibration1 : MotoHawk_lib/Calibration & Probing Blocks/motohawk_calibration  nam=[nam 'IncFiltC']  val=1.25  storage=Calibration  show_more=on  name_source=Use Parameter  data_type=Inherit from 'Default Value'  read_level=1  write_level=1  ovr_cals=on  view_as=Number  enum_struct={'Disabled', 'Enabled'}  vector_style=Wide Row  use_help_units=on  help='Filter time constant for a increasing signal.'  units='sec'  use_header_enum=off  row_header_enum={}  col_header_enum={}  use_min_max=off  min_val=-inf  max_val=inf  use_precision=off  precision=''  gain=1  offset=0  exp=1  use_mototune_group=on  mototune_group=grp_cal
  Out1 : Outport  InitialOutput=.005
  wires:
  motohawk_calibration1/1 -> Out1/1

== system BaseEngineController_LS_112/Foreground/Control/VirtualSensors/LoadBasedCalcs/Engine Steady-State Flag/Inc_DecFilterSelect3/DecreasingFilter ==
  Enable : EnablePort
  motohawk_calibration2 : MotoHawk_lib/Calibration & Probing Blocks/motohawk_calibration  nam=[nam 'DecFiltC']  val=1.25  storage=Calibration  show_more=on  name_source=Use Parameter  data_type=Inherit from 'Default Value'  read_level=1  write_level=1  ovr_cals=on  view_as=Number  enum_struct={'Disabled', 'Enabled'}  vector_style=Wide Row  use_help_units=on  help='Filter time constant for a decreasing signal.'  units='sec'  use_header_enum=off  row_header_enum={}  col_header_enum={}  use_min_max=off  min_val=-inf  max_val=inf  use_precision=off  precision=''  gain=1  offset=0  exp=1  use_mototune_group=on  mototune_group=grp_cal
  Out1 : Outport  InitialOutput=.005
  wires:
  motohawk_calibration2/1 -> Out1/1

== system BaseEngineController_LS_112/Foreground/Control/VirtualSensors/LoadBasedCalcs/Engine Steady-State Flag/Inc_DecFilterSelect3/IncreasingFilter ==
  Enable : EnablePort
  motohawk_calibration1 : MotoHawk_lib/Calibration & Probing Blocks/motohawk_calibration  nam=[nam 'IncFiltC']  val=1.25  storage=Calibration  show_more=on  name_source=Use Parameter  data_type=Inherit from 'Default Value'  read_level=1  write_level=1  ovr_cals=on  view_as=Number  enum_struct={'Disabled', 'Enabled'}  vector_style=Wide Row  use_help_units=on  help='Filter time constant for a increasing signal.'  units='sec'  use_header_enum=off  row_header_enum={}  col_header_enum={}  use_min_max=off  min_val=-inf  max_val=inf  use_precision=off  precision=''  gain=1  offset=0  exp=1  use_mototune_group=on  mototune_group=grp_cal
  Out1 : Outport  InitialOutput=.005
  wires:
  motohawk_calibration1/1 -> Out1/1

== system BaseEngineController_LS_112/Foreground/Control/Controller/Run/Fuel System Manager/Fuel Calculation/Calculate Fuel Flow/Calculate A/F Ratio ==
  Ethanol_xx [%] : Inport
  motohawk_table_1d : MotoHawk_lib/Lookup Tables/motohawk_table_1d  SystemSampleTime=-1  nam='DesAFRatio'  bp_nam=''  breakpoint_data=[0:10:100]  table_data=[14 14 14 14 14 14 14 14 14 14 14]  show_more=on  bp_data_type=Inherit from 'Breakpoint Data'  bp_storage=Constant  table_data_type=Inherit from 'Table Data'  storage=NonAdaptive  read_level=1  write_level=1  ovr_cals=on  use_help=on  help=''  bp_units='Ethanol%'  table_units='AFRatio'  use_min_max=on  bp_min_val=0  bp_max_val=100  min_val=0  max_val=20  use_precision=off  use_breakpoint=off  b_precision=''  b_gain=1  b_offset=0  b_exp=1  use_table=off  t_precision=''  t_gain=1  t_offset=0  t_exp=1  use_links=off  input_name=''  output_name=''  use_mototune_group=off  mototune_group=motohawk_vardec_path(gcb)
  Desired A/F Ratio : Outport
  wires:
  Ethanol_xx [%]/1 -> motohawk_table_1d/1
  motohawk_table_1d/1 -> Desired A/F Ratio/1

== system BaseEngineController_LS_112/Foreground/Control/Controller/Run/Fuel System Manager/Injector Manager/Delta TPS Transient Fueling/ECT Transient Fueling ==
  ECTIdx : Inport
  Enable : EnablePort
  motohawk_interpolation_1d : MotoHawk_lib/Lookup Tables/motohawk_interpolation_1d  nam='ECTTransFuelMult'  table_data=[1 1 1 1 1]  show_more=on  data_type=Inherit from 'Table Data'  storage=NonAdaptive  read_level=1  write_level=1  ovr_cals=on  use_help=on  help="'Transient fuel multiplier based on ECT.  Only engaged during transient fueling'"  units=''  use_min_max=off  min_val=-inf  max_val=inf  use_precision=off  precision=''  gain=1  offset=0  exp=1  use_links=off  prelookup_block=''  output_name=''  use_mototune_group=on  mototune_group=motohawk_vardec_path(gcb)
  Mult : Outport  OutputWhenDisabled=reset  InitialOutput=1
  wires:
  motohawk_interpolation_1d/1 -> Mult/1
  ECTIdx/1 -> motohawk_interpolation_1d/1

== system BaseEngineController_LS_112/Foreground/Control/Controller/Run/Fuel System Manager/Injector Manager/Delta TPS Transient Fueling/OXY Transient Fueling ==
  OXYIdx : Inport
  Enable : EnablePort
  motohawk_interpolation_1d : MotoHawk_lib/Lookup Tables/motohawk_interpolation_1d  nam='OXYTransFuelMult'  table_data=[1 1 1 1 1]  show_more=on  data_type=Inherit from 'Table Data'  storage=NonAdaptive  read_level=1  write_level=1  ovr_cals=on  use_help=on  help="'Transient fuel multiplier based on OXY.  Only engaged during transient fueling'"  units=''  use_min_max=on  min_val=-100  max_val=100  use_precision=off  precision=''  gain=1  offset=0  exp=1  use_links=off  prelookup_block=''  output_name=''  use_mototune_group=on  mototune_group=motohawk_vardec_path(gcb)
  Mult : Outport  OutputWhenDisabled=reset  InitialOutput=1
  wires:
  motohawk_interpolation_1d/1 -> Mult/1
  OXYIdx/1 -> motohawk_interpolation_1d/1

== system BaseEngineController_LS_112/Foreground/Control/Controller/Run/O2 Control/O2 PID Controller Bank A/Equivalence Ratio Perturbation/Hysteresis ==
  note: Hi & !Lo => Hi
      | Lo & !Hi => Lo
      | Otherwise, Hold
  Hi : Inport
  Lo : Inport  Port=2
  Combinatorial  Logic : CombinatorialLogic  TruthTable=[0 0;0 1;1 1;0 0]
  Demux : Demux  Outputs=2
  Mux : Mux  Inputs=2
  Switch1 : Switch  Threshold=0.5  SaturateOnIntegerOverflow=on  InputSameDT=on
  Unit Delay : UnitDelay  SampleTime=-1
  "Out (Lo=0, Hi=1)" : Outport
  wires:
  Mux/1 -> Combinatorial  Logic/1
  Combinatorial  Logic/1 -> Demux/1
  Demux/1 -> Switch1/1
  Demux/2 -> Switch1/2
  Unit Delay/1 -> Switch1/3
  Switch1/1 -> Unit Delay/1, "Out (Lo=0, Hi=1)"/1
  Hi/1 -> Mux/1
  Lo/1 -> Mux/2

== system BaseEngineController_LS_112/Foreground/Control/Controller/Run/O2 Control/O2 PID Controller Bank B/Equivalence Ratio Perturbation/Hysteresis ==
  note: Hi & !Lo => Hi
      | Lo & !Hi => Lo
      | Otherwise, Hold
  Hi : Inport
  Lo : Inport  Port=2
  Combinatorial  Logic : CombinatorialLogic  TruthTable=[0 0;0 1;1 1;0 0]
  Demux : Demux  Outputs=2
  Mux : Mux  Inputs=2
  Switch1 : Switch  Threshold=0.5  SaturateOnIntegerOverflow=on  InputSameDT=on
  Unit Delay : UnitDelay  SampleTime=-1
  "Out (Lo=0, Hi=1)" : Outport
  wires:
  Mux/1 -> Combinatorial  Logic/1
  Combinatorial  Logic/1 -> Demux/1
  Demux/1 -> Switch1/1
  Demux/2 -> Switch1/2
  Unit Delay/1 -> Switch1/3
  Switch1/1 -> Unit Delay/1, "Out (Lo=0, Hi=1)"/1
  Hi/1 -> Mux/1
  Lo/1 -> Mux/2

== system BaseEngineController_LS_112/Foreground/Control/Diagnostics/MISFIRE/MisfireDiagSub/MisfireDiagFunc/DetermineMisfire/DetermineCylinder ==
  ArrayIn : Inport
  Constant : Constant  Value=[1,2,3,4,5,6,7,8]
  MinMax : MinMax  Function=max
  Product : Product  RndMeth=Zero
  CylinderNum : Outport
  wires:
  ArrayIn/1 -> Product/1
  Constant/1 -> Product/2
  Product/1 -> MinMax/1
  MinMax/1 -> CylinderNum/1
